simulink model "KillerWhaleModel"  (R2020b)
settings: Solver=ode15s  StartTime=0.0  StopTime=10.0  MaxStep=0.01  RelTol=1e-3
model workspace: external: MATLAB File KillerWhaleParams.m (data not in the file)
undefined symbols (not defined in the file or in its folder): frontParams, rearParams, standParams, X, Y, Z
libraries: sm_lib x4076, nesl_utility x6
(part 6 of 62)

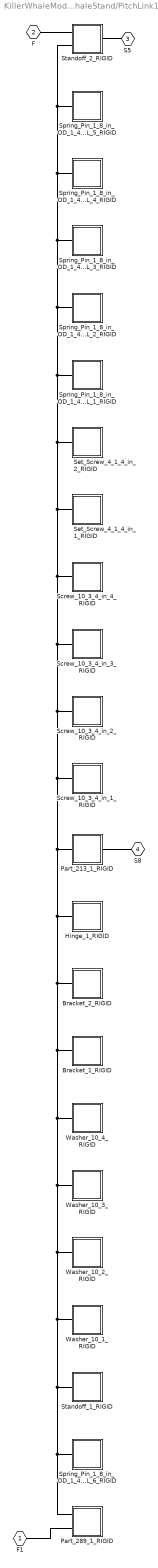
== system KillerWhaleModel/WhaleStand/PitchLink1_1 ==
  Bracket_1_RIGID : Subsystem
  Bracket_2_RIGID : Subsystem
  Hinge_1_RIGID : Subsystem
  Part_213_1_RIGID : Subsystem
  Part_289_1_RIGID : Subsystem
  Screw_10_3_4_in_1_RIGID : Subsystem
  Screw_10_3_4_in_2_RIGID : Subsystem
  Screw_10_3_4_in_3_RIGID : Subsystem
  Screw_10_3_4_in_4_RIGID : Subsystem
  Set_Screw_4_1_4_in_1_RIGID : Subsystem
  Set_Screw_4_1_4_in_2_RIGID : Subsystem
  Spring_Pin_1_8_in_OD_1_4_in_L_1_RIGID : Subsystem
  Spring_Pin_1_8_in_OD_1_4_in_L_2_RIGID : Subsystem
  Spring_Pin_1_8_in_OD_1_4_in_L_3_RIGID : Subsystem
  Spring_Pin_1_8_in_OD_1_4_in_L_4_RIGID : Subsystem
  Spring_Pin_1_8_in_OD_1_4_in_L_5_RIGID : Subsystem
  Spring_Pin_1_8_in_OD_1_4_in_L_6_RIGID : Subsystem
  Standoff_1_RIGID : Subsystem
  Standoff_2_RIGID : Subsystem
  Washer_10_1_RIGID : Subsystem
  Washer_10_2_RIGID : Subsystem
  Washer_10_3_RIGID : Subsystem
  Washer_10_4_RIGID : Subsystem
  F1 : PMIOPort  Side=Left
  F : PMIOPort  Port=2  Side=Right
  S5 : PMIOPort  Port=3  Side=Right
  S8 : PMIOPort  Port=4  Side=Right
  connections:
  Bracket_1_RIGID/LConn1 -- Part_289_1_RIGID/LConn1 -- Spring_Pin_1_8_in_OD_1_4_in_L_6_RIGID/LConn1 -- Standoff_1_RIGID/LConn1 -- Washer_10_1_RIGID/LConn1 -- Washer_10_2_RIGID/LConn1 -- Washer_10_3_RIGID/LConn1 -- Washer_10_4_RIGID/LConn1 -- Spring_Pin_1_8_in_OD_1_4_in_L_5_RIGID/LConn1 -- Standoff_2_RIGID/LConn2 -- Spring_Pin_1_8_in_OD_1_4_in_L_4_RIGID/LConn1 -- Spring_Pin_1_8_in_OD_1_4_in_L_3_RIGID/LConn1 -- Spring_Pin_1_8_in_OD_1_4_in_L_2_RIGID/LConn1 -- Spring_Pin_1_8_in_OD_1_4_in_L_1_RIGID/LConn1 -- Set_Screw_4_1_4_in_2_RIGID/LConn1 -- Set_Screw_4_1_4_in_1_RIGID/LConn1 -- Screw_10_3_4_in_4_RIGID/LConn1 -- Screw_10_3_4_in_3_RIGID/LConn1 -- Screw_10_3_4_in_2_RIGID/LConn1 -- Screw_10_3_4_in_1_RIGID/LConn1 -- Part_213_1_RIGID/LConn1 -- Hinge_1_RIGID/LConn1 -- Bracket_2_RIGID/LConn1
  Standoff_2_RIGID/LConn1 -- F/RConn1
  Part_289_1_RIGID/LConn2 -- F1/RConn1
  S5/RConn1 -- Standoff_2_RIGID/RConn1
  S8/RConn1 -- Part_213_1_RIGID/RConn1

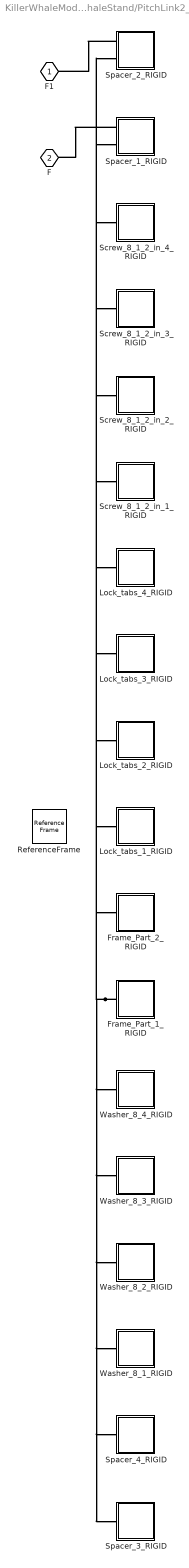
== system KillerWhaleModel/WhaleStand/PitchLink2_1 ==
  Frame_Part_1_RIGID : Subsystem
  Frame_Part_2_RIGID : Subsystem
  Lock_tabs_1_RIGID : Subsystem
  Lock_tabs_2_RIGID : Subsystem
  Lock_tabs_3_RIGID : Subsystem
  Lock_tabs_4_RIGID : Subsystem
  ReferenceFrame : sm_lib/Frames and Transforms/Reference Frame
  Screw_8_1_2_in_1_RIGID : Subsystem
  Screw_8_1_2_in_2_RIGID : Subsystem
  Screw_8_1_2_in_3_RIGID : Subsystem
  Screw_8_1_2_in_4_RIGID : Subsystem
  Spacer_1_RIGID : Subsystem
  Spacer_2_RIGID : Subsystem
  Spacer_3_RIGID : Subsystem
  Spacer_4_RIGID : Subsystem
  Washer_8_1_RIGID : Subsystem
  Washer_8_2_RIGID : Subsystem
  Washer_8_3_RIGID : Subsystem
  Washer_8_4_RIGID : Subsystem
  F1 : PMIOPort  Side=Right
  F : PMIOPort  Port=2  Side=Right
  connections:
  Frame_Part_1_RIGID/LConn1 -- Frame_Part_2_RIGID/LConn1 -- Lock_tabs_1_RIGID/LConn1 -- Lock_tabs_2_RIGID/LConn1 -- Lock_tabs_3_RIGID/LConn1 -- Lock_tabs_4_RIGID/LConn1 -- Screw_8_1_2_in_1_RIGID/LConn1 -- Screw_8_1_2_in_2_RIGID/LConn1 -- Screw_8_1_2_in_3_RIGID/LConn1 -- Screw_8_1_2_in_4_RIGID/LConn1 -- Spacer_1_RIGID/LConn2 -- Spacer_2_RIGID/LConn2 -- Spacer_3_RIGID/LConn1 -- Spacer_4_RIGID/LConn1 -- Washer_8_1_RIGID/LConn1 -- Washer_8_2_RIGID/LConn1 -- Washer_8_3_RIGID/LConn1 -- Washer_8_4_RIGID/LConn1
  Spacer_1_RIGID/LConn1 -- F/RConn1
  Spacer_2_RIGID/LConn1 -- F1/RConn1

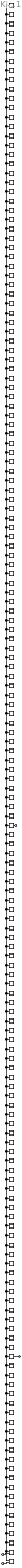
== system KillerWhaleModel/WhaleStand/PitchLink3_1 ==
  Bracket_1_RIGID : Subsystem
  Bracket_2_RIGID : Subsystem
  Bracket_3_RIGID : Subsystem
  Bracket_4_RIGID : Subsystem
  Hinge_1_RIGID : Subsystem
  Part_144_1_RIGID : Subsystem
  Part_145_1_RIGID : Subsystem
  Part_146_1_RIGID : Subsystem
  Part_147_1_RIGID : Subsystem
  Part_148_1_RIGID : Subsystem
  Part_149_1_RIGID : Subsystem
  Part_150_1_RIGID : Subsystem
  Part_151_1_RIGID : Subsystem
  Part_152_1_RIGID : Subsystem
  Part_153_1_RIGID : Subsystem
  Part_154_1_RIGID : Subsystem
  Part_155_1_RIGID : Subsystem
  Part_168_1_RIGID : Subsystem
  Part_169_1_RIGID : Subsystem
  Part_170_1_RIGID : Subsystem
  Part_171_1_RIGID : Subsystem
  Part_172_1_RIGID : Subsystem
  Part_173_1_RIGID : Subsystem
  Part_174_1_RIGID : Subsystem
  Part_175_1_RIGID : Subsystem
  Part_176_1_RIGID : Subsystem
  Part_177_1_RIGID : Subsystem
  Part_178_1_RIGID : Subsystem
  Part_179_1_RIGID : Subsystem
  Part_186_1_RIGID : Subsystem
  Part_187_1_RIGID : Subsystem
  Part_188_1_RIGID : Subsystem
  Part_190_1_RIGID : Subsystem
  Part_191_1_RIGID : Subsystem
  Part_192_1_RIGID : Subsystem
  Part_193_1_RIGID : Subsystem
  Part_194_1_RIGID : Subsystem
  Part_195_1_RIGID : Subsystem
  Part_196_1_RIGID : Subsystem
  Part_197_1_RIGID : Subsystem
  Part_318_1_RIGID : Subsystem
  Part_319_1_RIGID : Subsystem
  Part_322_1_RIGID : Subsystem
  Part_325_1_RIGID : Subsystem
  Part_328_1_RIGID : Subsystem
  Part_331_1_RIGID : Subsystem
  Part_334_1_RIGID : Subsystem
  Part_337_1_RIGID : Subsystem
  Part_340_1_RIGID : Subsystem
  Part_343_1_RIGID : Subsystem
  Part_346_1_RIGID : Subsystem
  Part_349_1_RIGID : Subsystem
  Part_360_1_RIGID : Subsystem
  Part_361_1_RIGID : Subsystem
  Part_362_1_RIGID : Subsystem
  Part_363_1_RIGID : Subsystem
  Part_364_1_RIGID : Subsystem
  Part_365_1_RIGID : Subsystem
  Part_366_1_RIGID : Subsystem
  Part_367_1_RIGID : Subsystem
  Part_368_1_RIGID : Subsystem
  Part_369_1_RIGID : Subsystem
  Part_370_1_RIGID : Subsystem
  Part_371_1_RIGID : Subsystem
  Part_372_1_RIGID : Subsystem
  Part_373_1_RIGID : Subsystem
  Part_374_1_RIGID : Subsystem
  Part_375_1_RIGID : Subsystem
  Part_380_1_RIGID : Subsystem
  Part_386_1_RIGID : Subsystem
  Part_387_1_RIGID : Subsystem
  Part_393_1_RIGID : Subsystem
  Part_399_1_RIGID : Subsystem
  Part_400_1_RIGID : Subsystem
  Part_406_1_RIGID : Subsystem
  Part_412_1_RIGID : Subsystem
  Part_413_1_RIGID : Subsystem
  Screw_10_3_4_in_10_RIGID : Subsystem
  Screw_10_3_4_in_11_RIGID : Subsystem
  Screw_10_3_4_in_12_RIGID : Subsystem
  Screw_10_3_4_in_13_RIGID : Subsystem
  Screw_10_3_4_in_14_RIGID : Subsystem
  Screw_10_3_4_in_15_RIGID : Subsystem
  Screw_10_3_4_in_16_RIGID : Subsystem
  Screw_10_3_4_in_17_RIGID : Subsystem
  Screw_10_3_4_in_18_RIGID : Subsystem
  Screw_10_3_4_in_19_RIGID : Subsystem
  Screw_10_3_4_in_1_RIGID : Subsystem
  Screw_10_3_4_in_20_RIGID : Subsystem
  Screw_10_3_4_in_2_RIGID : Subsystem
  Screw_10_3_4_in_3_RIGID : Subsystem
  Screw_10_3_4_in_4_RIGID : Subsystem
  Screw_10_3_4_in_5_RIGID : Subsystem
  Screw_10_3_4_in_6_RIGID : Subsystem
  Screw_10_3_4_in_7_RIGID : Subsystem
  Screw_10_3_4_in_8_RIGID : Subsystem
  Screw_10_3_4_in_9_RIGID : Subsystem
  Set_Screw_4_1_4_in_1_RIGID : Subsystem
  Set_Screw_4_1_4_in_2_RIGID : Subsystem
  Set_Screw_4_1_4_in_3_RIGID : Subsystem
  Set_Screw_4_1_4_in_4_RIGID : Subsystem
  Spring_Pin_1_8_in_OD_1_4_in_L_10_RIGID : Subsystem
  Spring_Pin_1_8_in_OD_1_4_in_L_11_RIGID : Subsystem
  Spring_Pin_1_8_in_OD_1_4_in_L_12_RIGID : Subsystem
  Spring_Pin_1_8_in_OD_1_4_in_L_13_RIGID : Subsystem
  Spring_Pin_1_8_in_OD_1_4_in_L_14_RIGID : Subsystem
  Spring_Pin_1_8_in_OD_1_4_in_L_15_RIGID : Subsystem
  Spring_Pin_1_8_in_OD_1_4_in_L_16_RIGID : Subsystem
  Spring_Pin_1_8_in_OD_1_4_in_L_17_RIGID : Subsystem
  Spring_Pin_1_8_in_OD_1_4_in_L_18_RIGID : Subsystem
  Spring_Pin_1_8_in_OD_1_4_in_L_19_RIGID : Subsystem
  Spring_Pin_1_8_in_OD_1_4_in_L_1_RIGID : Subsystem
  Spring_Pin_1_8_in_OD_1_4_in_L_20_RIGID : Subsystem
  Spring_Pin_1_8_in_OD_1_4_in_L_21_RIGID : Subsystem
  Spring_Pin_1_8_in_OD_1_4_in_L_22_RIGID : Subsystem
  Spring_Pin_1_8_in_OD_1_4_in_L_23_RIGID : Subsystem
  Spring_Pin_1_8_in_OD_1_4_in_L_24_RIGID : Subsystem
  Spring_Pin_1_8_in_OD_1_4_in_L_25_RIGID : Subsystem
  Spring_Pin_1_8_in_OD_1_4_in_L_26_RIGID : Subsystem
  Spring_Pin_1_8_in_OD_1_4_in_L_27_RIGID : Subsystem
  Spring_Pin_1_8_in_OD_1_4_in_L_28_RIGID : Subsystem
  Spring_Pin_1_8_in_OD_1_4_in_L_29_RIGID : Subsystem
  Spring_Pin_1_8_in_OD_1_4_in_L_2_RIGID : Subsystem
  Spring_Pin_1_8_in_OD_1_4_in_L_30_RIGID : Subsystem
  Spring_Pin_1_8_in_OD_1_4_in_L_31_RIGID : Subsystem
  Spring_Pin_1_8_in_OD_1_4_in_L_32_RIGID : Subsystem
  Spring_Pin_1_8_in_OD_1_4_in_L_33_RIGID : Subsystem
  Spring_Pin_1_8_in_OD_1_4_in_L_34_RIGID : Subsystem
  Spring_Pin_1_8_in_OD_1_4_in_L_35_RIGID : Subsystem
  Spring_Pin_1_8_in_OD_1_4_in_L_36_RIGID : Subsystem
  Spring_Pin_1_8_in_OD_1_4_in_L_37_RIGID : Subsystem
  Spring_Pin_1_8_in_OD_1_4_in_L_38_RIGID : Subsystem
  Spring_Pin_1_8_in_OD_1_4_in_L_39_RIGID : Subsystem
  Spring_Pin_1_8_in_OD_1_4_in_L_3_RIGID : Subsystem
  Spring_Pin_1_8_in_OD_1_4_in_L_40_RIGID : Subsystem
  Spring_Pin_1_8_in_OD_1_4_in_L_41_RIGID : Subsystem
  Spring_Pin_1_8_in_OD_1_4_in_L_4_RIGID : Subsystem
  Spring_Pin_1_8_in_OD_1_4_in_L_5_RIGID : Subsystem
  Spring_Pin_1_8_in_OD_1_4_in_L_6_RIGID : Subsystem
  Spring_Pin_1_8_in_OD_1_4_in_L_7_RIGID : Subsystem
  Spring_Pin_1_8_in_OD_1_4_in_L_8_RIGID : Subsystem
  Spring_Pin_1_8_in_OD_1_4_in_L_9_RIGID : Subsystem
  Washer_10_10_RIGID : Subsystem
  Washer_10_11_RIGID : Subsystem
  Washer_10_12_RIGID : Subsystem
  Washer_10_13_RIGID : Subsystem
  Washer_10_14_RIGID : Subsystem
  Washer_10_15_RIGID : Subsystem
  Washer_10_16_RIGID : Subsystem
  Washer_10_17_RIGID : Subsystem
  Washer_10_18_RIGID : Subsystem
  Washer_10_19_RIGID : Subsystem
  Washer_10_1_RIGID : Subsystem
  Washer_10_20_RIGID : Subsystem
  Washer_10_2_RIGID : Subsystem
  Washer_10_3_RIGID : Subsystem
  Washer_10_4_RIGID : Subsystem
  Washer_10_5_RIGID : Subsystem
  Washer_10_6_RIGID : Subsystem
  Washer_10_7_RIGID : Subsystem
  Washer_10_8_RIGID : Subsystem
  Washer_10_9_RIGID : Subsystem
  forward_torso_l_1_RIGID : Subsystem
  forward_torso_l_2_RIGID : Subsystem
  forward_torso_l_3_RIGID : Subsystem
  forward_torso_l_4_RIGID : Subsystem
  forward_torso_l_5_RIGID : Subsystem
  nut_1_RIGID : Subsystem
  F1 : PMIOPort  Side=Left
  S6 : PMIOPort  Port=2  Side=Left
  F : PMIOPort  Port=3  Side=Right
  S1 : PMIOPort  Port=4  Side=Right
  connections:
  Bracket_1_RIGID/LConn1 -- Part_150_1_RIGID/LConn1 -- Part_318_1_RIGID/LConn1 -- Part_346_1_RIGID/LConn1 -- Washer_10_7_RIGID/LConn1 -- Washer_10_8_RIGID/LConn1 -- Washer_10_9_RIGID/LConn1 -- forward_torso_l_1_RIGID/LConn1 -- forward_torso_l_2_RIGID/LConn1 -- forward_torso_l_3_RIGID/LConn1 -- forward_torso_l_4_RIGID/LConn1 -- forward_torso_l_5_RIGID/LConn1 -- nut_1_RIGID/LConn1 -- Washer_10_5_RIGID/LConn1 -- Washer_10_6_RIGID/LConn1 -- Washer_10_4_RIGID/LConn1 -- Washer_10_3_RIGID/LConn1 -- Washer_10_2_RIGID/LConn1 -- Washer_10_20_RIGID/LConn1 -- Washer_10_1_RIGID/LConn1 -- Washer_10_19_RIGID/LConn1 -- Washer_10_18_RIGID/LConn1 -- Washer_10_17_RIGID/LConn1 -- Washer_10_16_RIGID/LConn1 -- Washer_10_15_RIGID/LConn1 -- Washer_10_14_RIGID/LConn1 -- Washer_10_13_RIGID/LConn1 -- Washer_10_12_RIGID/LConn1 -- Washer_10_11_RIGID/LConn1 -- Washer_10_10_RIGID/LConn1 -- Spring_Pin_1_8_in_OD_1_4_in_L_9_RIGID/LConn1 -- Spring_Pin_1_8_in_OD_1_4_in_L_8_RIGID/LConn1 -- Spring_Pin_1_8_in_OD_1_4_in_L_7_RIGID/LConn1 -- Spring_Pin_1_8_in_OD_1_4_in_L_6_RIGID/LConn1 -- Spring_Pin_1_8_in_OD_1_4_in_L_5_RIGID/LConn1 -- Spring_Pin_1_8_in_OD_1_4_in_L_4_RIGID/LConn1 -- Spring_Pin_1_8_in_OD_1_4_in_L_41_RIGID/LConn1 -- Spring_Pin_1_8_in_OD_1_4_in_L_40_RIGID/LConn1 -- Spring_Pin_1_8_in_OD_1_4_in_L_3_RIGID/LConn1 -- Spring_Pin_1_8_in_OD_1_4_in_L_39_RIGID/LConn1 -- Spring_Pin_1_8_in_OD_1_4_in_L_38_RIGID/LConn1 -- Spring_Pin_1_8_in_OD_1_4_in_L_37_RIGID/LConn1 -- Spring_Pin_1_8_in_OD_1_4_in_L_36_RIGID/LConn1 -- Spring_Pin_1_8_in_OD_1_4_in_L_35_RIGID/LConn1 -- Spring_Pin_1_8_in_OD_1_4_in_L_34_RIGID/LConn1 -- Spring_Pin_1_8_in_OD_1_4_in_L_33_RIGID/LConn1 -- Spring_Pin_1_8_in_OD_1_4_in_L_32_RIGID/LConn1 -- Spring_Pin_1_8_in_OD_1_4_in_L_31_RIGID/LConn1 -- Spring_Pin_1_8_in_OD_1_4_in_L_30_RIGID/LConn1 -- Spring_Pin_1_8_in_OD_1_4_in_L_2_RIGID/LConn1 -- Spring_Pin_1_8_in_OD_1_4_in_L_29_RIGID/LConn1 -- Spring_Pin_1_8_in_OD_1_4_in_L_28_RIGID/LConn1 -- Spring_Pin_1_8_in_OD_1_4_in_L_27_RIGID/LConn1 -- Spring_Pin_1_8_in_OD_1_4_in_L_26_RIGID/LConn1 -- Spring_Pin_1_8_in_OD_1_4_in_L_25_RIGID/LConn1 -- Spring_Pin_1_8_in_OD_1_4_in_L_24_RIGID/LConn1 -- Spring_Pin_1_8_in_OD_1_4_in_L_23_RIGID/LConn1 -- Spring_Pin_1_8_in_OD_1_4_in_L_22_RIGID/LConn1 -- Spring_Pin_1_8_in_OD_1_4_in_L_21_RIGID/LConn1 -- Spring_Pin_1_8_in_OD_1_4_in_L_20_RIGID/LConn1 -- Spring_Pin_1_8_in_OD_1_4_in_L_1_RIGID/LConn1 -- Spring_Pin_1_8_in_OD_1_4_in_L_19_RIGID/LConn1 -- Spring_Pin_1_8_in_OD_1_4_in_L_18_RIGID/LConn1 -- Spring_Pin_1_8_in_OD_1_4_in_L_17_RIGID/LConn1 -- Spring_Pin_1_8_in_OD_1_4_in_L_16_RIGID/LConn1 -- Spring_Pin_1_8_in_OD_1_4_in_L_15_RIGID/LConn1 -- Spring_Pin_1_8_in_OD_1_4_in_L_14_RIGID/LConn1 -- Spring_Pin_1_8_in_OD_1_4_in_L_13_RIGID/LConn1 -- Spring_Pin_1_8_in_OD_1_4_in_L_12_RIGID/LConn1 -- Spring_Pin_1_8_in_OD_1_4_in_L_11_RIGID/LConn1 -- Spring_Pin_1_8_in_OD_1_4_in_L_10_RIGID/LConn1 -- Set_Screw_4_1_4_in_4_RIGID/LConn1 -- Set_Screw_4_1_4_in_3_RIGID/LConn1 -- Set_Screw_4_1_4_in_2_RIGID/LConn1 -- Set_Screw_4_1_4_in_1_RIGID/LConn1 -- Screw_10_3_4_in_9_RIGID/LConn1 -- Screw_10_3_4_in_8_RIGID/LConn1 -- Screw_10_3_4_in_7_RIGID/LConn1 -- Screw_10_3_4_in_6_RIGID/LConn1 -- Screw_10_3_4_in_5_RIGID/LConn1 -- Screw_10_3_4_in_4_RIGID/LConn1 -- Screw_10_3_4_in_3_RIGID/LConn1 -- Screw_10_3_4_in_2_RIGID/LConn1 -- Screw_10_3_4_in_20_RIGID/LConn1 -- Screw_10_3_4_in_1_RIGID/LConn1 -- Screw_10_3_4_in_19_RIGID/LConn1 -- Screw_10_3_4_in_18_RIGID/LConn1 -- Screw_10_3_4_in_17_RIGID/LConn1 -- Screw_10_3_4_in_16_RIGID/LConn1 -- Screw_10_3_4_in_15_RIGID/LConn1 -- Screw_10_3_4_in_14_RIGID/LConn1 -- Screw_10_3_4_in_13_RIGID/LConn1 -- Screw_10_3_4_in_12_RIGID/LConn1 -- Screw_10_3_4_in_11_RIGID/LConn1 -- Screw_10_3_4_in_10_RIGID/LConn1 -- Part_413_1_RIGID/LConn1 -- Part_412_1_RIGID/LConn1 -- Part_406_1_RIGID/LConn1 -- Part_400_1_RIGID/LConn1 -- Part_399_1_RIGID/LConn1 -- Part_393_1_RIGID/LConn1 -- Part_387_1_RIGID/LConn1 -- Part_386_1_RIGID/LConn1 -- Part_380_1_RIGID/LConn1 -- Part_375_1_RIGID/LConn1 -- Part_374_1_RIGID/LConn1 -- Part_373_1_RIGID/LConn1 -- Part_372_1_RIGID/LConn1 -- Part_371_1_RIGID/LConn1 -- Part_370_1_RIGID/LConn1 -- Part_369_1_RIGID/LConn1 -- Part_368_1_RIGID/LConn1 -- Part_367_1_RIGID/LConn1 -- Part_366_1_RIGID/LConn1 -- Part_365_1_RIGID/LConn1 -- Part_364_1_RIGID/LConn1 -- Part_363_1_RIGID/LConn1 -- Part_362_1_RIGID/LConn1 -- Part_361_1_RIGID/LConn1 -- Part_360_1_RIGID/LConn1 -- Part_349_1_RIGID/LConn1 -- Part_343_1_RIGID/LConn1 -- Part_340_1_RIGID/LConn1 -- Part_337_1_RIGID/LConn1 -- Part_334_1_RIGID/LConn1 -- Part_331_1_RIGID/LConn1 -- Part_328_1_RIGID/LConn1 -- Part_325_1_RIGID/LConn1 -- Part_322_1_RIGID/LConn1 -- Part_319_1_RIGID/LConn1 -- Part_197_1_RIGID/LConn1 -- Part_196_1_RIGID/LConn1 -- Part_195_1_RIGID/LConn1 -- Part_194_1_RIGID/LConn1 -- Part_193_1_RIGID/LConn1 -- Part_192_1_RIGID/LConn1 -- Part_191_1_RIGID/LConn1 -- Part_190_1_RIGID/LConn1 -- Part_188_1_RIGID/LConn1 -- Part_187_1_RIGID/LConn1 -- Part_186_1_RIGID/LConn1 -- Part_179_1_RIGID/LConn1 -- Part_178_1_RIGID/LConn1 -- Part_177_1_RIGID/LConn1 -- Part_176_1_RIGID/LConn1 -- Part_175_1_RIGID/LConn1 -- Part_174_1_RIGID/LConn1 -- Part_173_1_RIGID/LConn1 -- Part_172_1_RIGID/LConn1 -- Part_171_1_RIGID/LConn1 -- Part_170_1_RIGID/LConn1 -- Part_169_1_RIGID/LConn1 -- Part_168_1_RIGID/LConn1 -- Part_155_1_RIGID/LConn1 -- Part_154_1_RIGID/LConn1 -- Part_153_1_RIGID/LConn1 -- Part_152_1_RIGID/LConn1 -- Part_151_1_RIGID/LConn1 -- Part_149_1_RIGID/LConn1 -- Part_148_1_RIGID/LConn1 -- Part_147_1_RIGID/LConn1 -- Part_146_1_RIGID/LConn1 -- Part_145_1_RIGID/LConn1 -- Part_144_1_RIGID/LConn1 -- Hinge_1_RIGID/LConn1 -- Bracket_4_RIGID/LConn1 -- Bracket_3_RIGID/LConn1 -- Bracket_2_RIGID/LConn1
  Part_150_1_RIGID/LConn2 -- F/RConn1
  Part_318_1_RIGID/LConn2 -- F1/RConn1
  S1/RConn1 -- Part_149_1_RIGID/RConn1
  S6/RConn1 -- Part_387_1_RIGID/RConn1

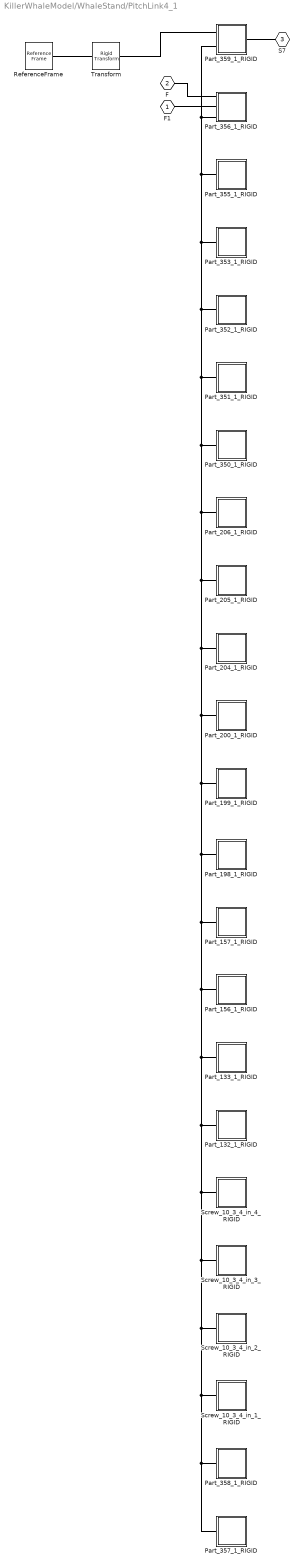
== system KillerWhaleModel/WhaleStand/PitchLink4_1 ==
  Part_132_1_RIGID : Subsystem
  Part_133_1_RIGID : Subsystem
  Part_156_1_RIGID : Subsystem
  Part_157_1_RIGID : Subsystem
  Part_198_1_RIGID : Subsystem
  Part_199_1_RIGID : Subsystem
  Part_200_1_RIGID : Subsystem
  Part_204_1_RIGID : Subsystem
  Part_205_1_RIGID : Subsystem
  Part_206_1_RIGID : Subsystem
  Part_350_1_RIGID : Subsystem
  Part_351_1_RIGID : Subsystem
  Part_352_1_RIGID : Subsystem
  Part_353_1_RIGID : Subsystem
  Part_355_1_RIGID : Subsystem
  Part_356_1_RIGID : Subsystem
  Part_357_1_RIGID : Subsystem
  Part_358_1_RIGID : Subsystem
  Part_359_1_RIGID : Subsystem
  ReferenceFrame : sm_lib/Frames and Transforms/Reference Frame
  Screw_10_3_4_in_1_RIGID : Subsystem
  Screw_10_3_4_in_2_RIGID : Subsystem
  Screw_10_3_4_in_3_RIGID : Subsystem
  Screw_10_3_4_in_4_RIGID : Subsystem
  Transform : sm_lib/Frames and Transforms/Rigid Transform  TranslationMethod=Cartesian  TranslationStandardOffset=0  TranslationLengthUnit=in  TranslationStandardAxis=+Z  TranslationCartesianOffset=standParams.RigidTransform(241).translation  TranslationROffset=0  TranslationROffsetUnits=m  TranslationZOffset=0  TranslationZOffsetUnits=m  TranslationThetaOffset=0  TranslationThetaOffsetUnits=deg  RotationMethod=ArbitraryAxis  RotationAngleUnits=rad  RotationStandardAxis=+Z  RotationAngle=standParams.RigidTransform(241).angle  RotationArbitraryAxis=standParams.RigidTransform(241).axis  FollAlignAxisA=+X  BaseAlignAxisA=+Y  FollAlignAxisB=+Y  BaseAlignAxisB=+Z  RotationSequenceAxes=FollowerAxes  RotationSequence=XYX  RotationSequenceAngles=[0 0 0]  RotationSequenceAnglesUnits=deg  RotationMatrix=[1 0 0; 0 1 0; 0 0 1]
  F1 : PMIOPort  Side=Left
  F : PMIOPort  Port=2  Side=Left
  S7 : PMIOPort  Port=3  Side=Right
  connections:
  Part_132_1_RIGID/LConn1 -- Part_357_1_RIGID/LConn1 -- Part_358_1_RIGID/LConn1 -- Screw_10_3_4_in_1_RIGID/LConn1 -- Screw_10_3_4_in_2_RIGID/LConn1 -- Screw_10_3_4_in_3_RIGID/LConn1 -- Screw_10_3_4_in_4_RIGID/LConn1 -- Part_356_1_RIGID/LConn3 -- Part_359_1_RIGID/LConn2 -- Part_355_1_RIGID/LConn1 -- Part_353_1_RIGID/LConn1 -- Part_352_1_RIGID/LConn1 -- Part_351_1_RIGID/LConn1 -- Part_350_1_RIGID/LConn1 -- Part_206_1_RIGID/LConn1 -- Part_205_1_RIGID/LConn1 -- Part_204_1_RIGID/LConn1 -- Part_200_1_RIGID/LConn1 -- Part_199_1_RIGID/LConn1 -- Part_198_1_RIGID/LConn1 -- Part_157_1_RIGID/LConn1 -- Part_156_1_RIGID/LConn1 -- Part_133_1_RIGID/LConn1
  Part_356_1_RIGID/LConn1 -- F/RConn1
  Part_356_1_RIGID/LConn2 -- F1/RConn1
  Part_359_1_RIGID/LConn1 -- Transform/RConn1
  ReferenceFrame/RConn1 -- Transform/LConn1
  S7/RConn1 -- Part_359_1_RIGID/RConn1

== system KillerWhaleModel/HeadLinkage/HeadLink1_1/Bracket_1_RIGID ==
  ReferenceFrame : sm_lib/Frames and Transforms/Reference Frame
  Solid : sm_lib/Body Elements/File Solid  ExtGeomFileName=Bracket13.step  UnitType=FromFile  ExtGeomFileUnits=m  StepReaderType=HEX  ExportConvexHullGeometry=off  InertiaType=Custom  Mass=frontParams.Solid(20).mass  MassUnits=lbm  CenterOfMass=frontParams.Solid(20).CoM  CenterOfMassUnits=in  MomentsOfInertia=frontParams.Solid(20).MoI  MomentsOfInertiaUnits=lbm*in^2  ProductsOfInertia=frontParams.Solid(20).PoI  ProductsOfInertiaUnits=lbm*in^2  BasedOnType=DensityFromFile  Density=1000  DensityUnits=kg/m^3  DoExposeReferenceFrame=on  SerializedFrames=<Frames/>  GraphicType=FromGeometry  MarkerShape=Sphere  MarkerSize=10  GraphicVisPropType=SimpleVisualProperties  GraphicDiffuseColor=frontParams.Solid(20).color  GraphicSpecularColor=[0.5 0.5 0.5 1.0]  GraphicAmbientColor=[0.15 0.15 0.15 1.0]  GraphicEmissiveColor=[0.0 0.0 0.0 1.0]  GraphicShininess=75  GraphicOpacity=frontParams.Solid(20).opacity
  Transform : sm_lib/Frames and Transforms/Rigid Transform  TranslationMethod=Cartesian  TranslationStandardOffset=0  TranslationLengthUnit=in  TranslationStandardAxis=+Z  TranslationCartesianOffset=frontParams.RigidTransform(33).translation  TranslationROffset=0  TranslationROffsetUnits=m  TranslationZOffset=0  TranslationZOffsetUnits=m  TranslationThetaOffset=0  TranslationThetaOffsetUnits=deg  RotationMethod=ArbitraryAxis  RotationAngleUnits=rad  RotationStandardAxis=+Z  RotationAngle=frontParams.RigidTransform(33).angle  RotationArbitraryAxis=frontParams.RigidTransform(33).axis  FollAlignAxisA=+X  BaseAlignAxisA=+Y  FollAlignAxisB=+Y  BaseAlignAxisB=+Z  RotationSequenceAxes=FollowerAxes  RotationSequence=XYX  RotationSequenceAngles=[0 0 0]  RotationSequenceAnglesUnits=deg  RotationMatrix=[1 0 0; 0 1 0; 0 0 1]
  G : PMIOPort  Side=Left
  connections:
  ReferenceFrame/RConn1 -- Solid/RConn1 -- Transform/RConn1
  Transform/LConn1 -- G/RConn1

== system KillerWhaleModel/HeadLinkage/HeadLink1_1/Bracket_2_RIGID ==
  ReferenceFrame : sm_lib/Frames and Transforms/Reference Frame
  Solid : sm_lib/Body Elements/File Solid  ExtGeomFileName=Bracket14.step  UnitType=FromFile  ExtGeomFileUnits=m  StepReaderType=HEX  ExportConvexHullGeometry=off  InertiaType=Custom  Mass=frontParams.Solid(52).mass  MassUnits=lbm  CenterOfMass=frontParams.Solid(52).CoM  CenterOfMassUnits=in  MomentsOfInertia=frontParams.Solid(52).MoI  MomentsOfInertiaUnits=lbm*in^2  ProductsOfInertia=frontParams.Solid(52).PoI  ProductsOfInertiaUnits=lbm*in^2  BasedOnType=DensityFromFile  Density=1000  DensityUnits=kg/m^3  DoExposeReferenceFrame=on  SerializedFrames=<Frames/>  GraphicType=FromGeometry  MarkerShape=Sphere  MarkerSize=10  GraphicVisPropType=SimpleVisualProperties  GraphicDiffuseColor=frontParams.Solid(52).color  GraphicSpecularColor=[0.5 0.5 0.5 1.0]  GraphicAmbientColor=[0.15 0.15 0.15 1.0]  GraphicEmissiveColor=[0.0 0.0 0.0 1.0]  GraphicShininess=75  GraphicOpacity=frontParams.Solid(52).opacity
  Transform : sm_lib/Frames and Transforms/Rigid Transform  TranslationMethod=Cartesian  TranslationStandardOffset=0  TranslationLengthUnit=in  TranslationStandardAxis=+Z  TranslationCartesianOffset=frontParams.RigidTransform(65).translation  TranslationROffset=0  TranslationROffsetUnits=m  TranslationZOffset=0  TranslationZOffsetUnits=m  TranslationThetaOffset=0  TranslationThetaOffsetUnits=deg  RotationMethod=ArbitraryAxis  RotationAngleUnits=rad  RotationStandardAxis=+Z  RotationAngle=frontParams.RigidTransform(65).angle  RotationArbitraryAxis=frontParams.RigidTransform(65).axis  FollAlignAxisA=+X  BaseAlignAxisA=+Y  FollAlignAxisB=+Y  BaseAlignAxisB=+Z  RotationSequenceAxes=FollowerAxes  RotationSequence=XYX  RotationSequenceAngles=[0 0 0]  RotationSequenceAnglesUnits=deg  RotationMatrix=[1 0 0; 0 1 0; 0 0 1]
  G : PMIOPort  Side=Left
  connections:
  ReferenceFrame/RConn1 -- Solid/RConn1 -- Transform/RConn1
  Transform/LConn1 -- G/RConn1

== system KillerWhaleModel/HeadLinkage/HeadLink1_1/Hinge_1_RIGID ==
  ReferenceFrame : sm_lib/Frames and Transforms/Reference Frame
  Solid : sm_lib/Body Elements/File Solid  ExtGeomFileName=Hinge6.step  UnitType=FromFile  ExtGeomFileUnits=m  StepReaderType=HEX  ExportConvexHullGeometry=off  InertiaType=Custom  Mass=frontParams.Solid(3).mass  MassUnits=lbm  CenterOfMass=frontParams.Solid(3).CoM  CenterOfMassUnits=in  MomentsOfInertia=frontParams.Solid(3).MoI  MomentsOfInertiaUnits=lbm*in^2  ProductsOfInertia=frontParams.Solid(3).PoI  ProductsOfInertiaUnits=lbm*in^2  BasedOnType=DensityFromFile  Density=1000  DensityUnits=kg/m^3  DoExposeReferenceFrame=on  SerializedFrames=<Frames/>  GraphicType=FromGeometry  MarkerShape=Sphere  MarkerSize=10  GraphicVisPropType=SimpleVisualProperties  GraphicDiffuseColor=frontParams.Solid(3).color  GraphicSpecularColor=[0.5 0.5 0.5 1.0]  GraphicAmbientColor=[0.15 0.15 0.15 1.0]  GraphicEmissiveColor=[0.0 0.0 0.0 1.0]  GraphicShininess=75  GraphicOpacity=frontParams.Solid(3).opacity
  Transform : sm_lib/Frames and Transforms/Rigid Transform  TranslationMethod=Cartesian  TranslationStandardOffset=0  TranslationLengthUnit=in  TranslationStandardAxis=+Z  TranslationCartesianOffset=frontParams.RigidTransform(16).translation  TranslationROffset=0  TranslationROffsetUnits=m  TranslationZOffset=0  TranslationZOffsetUnits=m  TranslationThetaOffset=0  TranslationThetaOffsetUnits=deg  RotationMethod=ArbitraryAxis  RotationAngleUnits=rad  RotationStandardAxis=+Z  RotationAngle=frontParams.RigidTransform(16).angle  RotationArbitraryAxis=frontParams.RigidTransform(16).axis  FollAlignAxisA=+X  BaseAlignAxisA=+Y  FollAlignAxisB=+Y  BaseAlignAxisB=+Z  RotationSequenceAxes=FollowerAxes  RotationSequence=XYX  RotationSequenceAngles=[0 0 0]  RotationSequenceAnglesUnits=deg  RotationMatrix=[1 0 0; 0 1 0; 0 0 1]
  G : PMIOPort  Side=Left
  connections:
  ReferenceFrame/RConn1 -- Solid/RConn1 -- Transform/RConn1
  Transform/LConn1 -- G/RConn1

== system KillerWhaleModel/HeadLinkage/HeadLink1_1/Part_1_1_RIGID ==
  ReferenceFrame : sm_lib/Frames and Transforms/Reference Frame
  Solid : sm_lib/Body Elements/File Solid  ExtGeomFileName=Part 111.step  UnitType=FromFile  ExtGeomFileUnits=m  StepReaderType=HEX  ExportConvexHullGeometry=off  InertiaType=Custom  Mass=frontParams.Solid(50).mass  MassUnits=lbm  CenterOfMass=frontParams.Solid(50).CoM  CenterOfMassUnits=in  MomentsOfInertia=frontParams.Solid(50).MoI  MomentsOfInertiaUnits=lbm*in^2  ProductsOfInertia=frontParams.Solid(50).PoI  ProductsOfInertiaUnits=lbm*in^2  BasedOnType=DensityFromFile  Density=1000  DensityUnits=kg/m^3  DoExposeReferenceFrame=on  SerializedFrames=<Frames/>  GraphicType=FromGeometry  MarkerShape=Sphere  MarkerSize=10  GraphicVisPropType=SimpleVisualProperties  GraphicDiffuseColor=frontParams.Solid(50).color  GraphicSpecularColor=[0.5 0.5 0.5 1.0]  GraphicAmbientColor=[0.15 0.15 0.15 1.0]  GraphicEmissiveColor=[0.0 0.0 0.0 1.0]  GraphicShininess=75  GraphicOpacity=frontParams.Solid(50).opacity
  Transform : sm_lib/Frames and Transforms/Rigid Transform  TranslationMethod=Cartesian  TranslationStandardOffset=0  TranslationLengthUnit=in  TranslationStandardAxis=+Z  TranslationCartesianOffset=frontParams.RigidTransform(63).translation  TranslationROffset=0  TranslationROffsetUnits=m  TranslationZOffset=0  TranslationZOffsetUnits=m  TranslationThetaOffset=0  TranslationThetaOffsetUnits=deg  RotationMethod=ArbitraryAxis  RotationAngleUnits=rad  RotationStandardAxis=+Z  RotationAngle=frontParams.RigidTransform(63).angle  RotationArbitraryAxis=frontParams.RigidTransform(63).axis  FollAlignAxisA=+X  BaseAlignAxisA=+Y  FollAlignAxisB=+Y  BaseAlignAxisB=+Z  RotationSequenceAxes=FollowerAxes  RotationSequence=XYX  RotationSequenceAngles=[0 0 0]  RotationSequenceAnglesUnits=deg  RotationMatrix=[1 0 0; 0 1 0; 0 0 1]
  G : PMIOPort  Side=Left
  connections:
  ReferenceFrame/RConn1 -- Solid/RConn1 -- Transform/RConn1
  Transform/LConn1 -- G/RConn1

== system KillerWhaleModel/HeadLinkage/HeadLink1_1/Part_1_2_RIGID ==
  ReferenceFrame : sm_lib/Frames and Transforms/Reference Frame
  Solid : sm_lib/Body Elements/File Solid  ExtGeomFileName=Part 110.step  UnitType=FromFile  ExtGeomFileUnits=m  StepReaderType=HEX  ExportConvexHullGeometry=off  InertiaType=Custom  Mass=frontParams.Solid(12).mass  MassUnits=lbm  CenterOfMass=frontParams.Solid(12).CoM  CenterOfMassUnits=in  MomentsOfInertia=frontParams.Solid(12).MoI  MomentsOfInertiaUnits=lbm*in^2  ProductsOfInertia=frontParams.Solid(12).PoI  ProductsOfInertiaUnits=lbm*in^2  BasedOnType=DensityFromFile  Density=1000  DensityUnits=kg/m^3  DoExposeReferenceFrame=on  SerializedFrames=<Frames/>  GraphicType=FromGeometry  MarkerShape=Sphere  MarkerSize=10  GraphicVisPropType=SimpleVisualProperties  GraphicDiffuseColor=frontParams.Solid(12).color  GraphicSpecularColor=[0.5 0.5 0.5 1.0]  GraphicAmbientColor=[0.15 0.15 0.15 1.0]  GraphicEmissiveColor=[0.0 0.0 0.0 1.0]  GraphicShininess=75  GraphicOpacity=frontParams.Solid(12).opacity
  Transform : sm_lib/Frames and Transforms/Rigid Transform  TranslationMethod=Cartesian  TranslationStandardOffset=0  TranslationLengthUnit=in  TranslationStandardAxis=+Z  TranslationCartesianOffset=frontParams.RigidTransform(25).translation  TranslationROffset=0  TranslationROffsetUnits=m  TranslationZOffset=0  TranslationZOffsetUnits=m  TranslationThetaOffset=0  TranslationThetaOffsetUnits=deg  RotationMethod=ArbitraryAxis  RotationAngleUnits=rad  RotationStandardAxis=+Z  RotationAngle=frontParams.RigidTransform(25).angle  RotationArbitraryAxis=frontParams.RigidTransform(25).axis  FollAlignAxisA=+X  BaseAlignAxisA=+Y  FollAlignAxisB=+Y  BaseAlignAxisB=+Z  RotationSequenceAxes=FollowerAxes  RotationSequence=XYX  RotationSequenceAngles=[0 0 0]  RotationSequenceAnglesUnits=deg  RotationMatrix=[1 0 0; 0 1 0; 0 0 1]
  G : PMIOPort  Side=Left
  connections:
  ReferenceFrame/RConn1 -- Solid/RConn1 -- Transform/RConn1
  Transform/LConn1 -- G/RConn1

== system KillerWhaleModel/HeadLinkage/HeadLink1_1/Part_2_1_RIGID ==
  ReferenceFrame : sm_lib/Frames and Transforms/Reference Frame
  Solid : sm_lib/Body Elements/File Solid  ExtGeomFileName=Part 28.step  UnitType=FromFile  ExtGeomFileUnits=m  StepReaderType=HEX  ExportConvexHullGeometry=off  InertiaType=Custom  Mass=frontParams.Solid(36).mass  MassUnits=lbm  CenterOfMass=frontParams.Solid(36).CoM  CenterOfMassUnits=in  MomentsOfInertia=frontParams.Solid(36).MoI  MomentsOfInertiaUnits=lbm*in^2  ProductsOfInertia=frontParams.Solid(36).PoI  ProductsOfInertiaUnits=lbm*in^2  BasedOnType=DensityFromFile  Density=1000  DensityUnits=kg/m^3  DoExposeReferenceFrame=on  SerializedFrames=<Frames/>  GraphicType=FromGeometry  MarkerShape=Sphere  MarkerSize=10  GraphicVisPropType=SimpleVisualProperties  GraphicDiffuseColor=frontParams.Solid(36).color  GraphicSpecularColor=[0.5 0.5 0.5 1.0]  GraphicAmbientColor=[0.15 0.15 0.15 1.0]  GraphicEmissiveColor=[0.0 0.0 0.0 1.0]  GraphicShininess=75  GraphicOpacity=frontParams.Solid(36).opacity
  Transform : sm_lib/Frames and Transforms/Rigid Transform  TranslationMethod=Cartesian  TranslationStandardOffset=0  TranslationLengthUnit=in  TranslationStandardAxis=+Z  TranslationCartesianOffset=frontParams.RigidTransform(49).translation  TranslationROffset=0  TranslationROffsetUnits=m  TranslationZOffset=0  TranslationZOffsetUnits=m  TranslationThetaOffset=0  TranslationThetaOffsetUnits=deg  RotationMethod=ArbitraryAxis  RotationAngleUnits=rad  RotationStandardAxis=+Z  RotationAngle=frontParams.RigidTransform(49).angle  RotationArbitraryAxis=frontParams.RigidTransform(49).axis  FollAlignAxisA=+X  BaseAlignAxisA=+Y  FollAlignAxisB=+Y  BaseAlignAxisB=+Z  RotationSequenceAxes=FollowerAxes  RotationSequence=XYX  RotationSequenceAngles=[0 0 0]  RotationSequenceAnglesUnits=deg  RotationMatrix=[1 0 0; 0 1 0; 0 0 1]
  G : PMIOPort  Side=Left
  connections:
  ReferenceFrame/RConn1 -- Solid/RConn1 -- Transform/RConn1
  Transform/LConn1 -- G/RConn1

== system KillerWhaleModel/HeadLinkage/HeadLink1_1/Part_2_2_RIGID ==
  ReferenceFrame : sm_lib/Frames and Transforms/Reference Frame
  Solid : sm_lib/Body Elements/File Solid  ExtGeomFileName=Part 27.step  UnitType=FromFile  ExtGeomFileUnits=m  StepReaderType=HEX  ExportConvexHullGeometry=off  InertiaType=Custom  Mass=frontParams.Solid(51).mass  MassUnits=lbm  CenterOfMass=frontParams.Solid(51).CoM  CenterOfMassUnits=in  MomentsOfInertia=frontParams.Solid(51).MoI  MomentsOfInertiaUnits=lbm*in^2  ProductsOfInertia=frontParams.Solid(51).PoI  ProductsOfInertiaUnits=lbm*in^2  BasedOnType=DensityFromFile  Density=1000  DensityUnits=kg/m^3  DoExposeReferenceFrame=on  SerializedFrames=<Frames/>  GraphicType=FromGeometry  MarkerShape=Sphere  MarkerSize=10  GraphicVisPropType=SimpleVisualProperties  GraphicDiffuseColor=frontParams.Solid(51).color  GraphicSpecularColor=[0.5 0.5 0.5 1.0]  GraphicAmbientColor=[0.15 0.15 0.15 1.0]  GraphicEmissiveColor=[0.0 0.0 0.0 1.0]  GraphicShininess=75  GraphicOpacity=frontParams.Solid(51).opacity
  Transform : sm_lib/Frames and Transforms/Rigid Transform  TranslationMethod=Cartesian  TranslationStandardOffset=0  TranslationLengthUnit=in  TranslationStandardAxis=+Z  TranslationCartesianOffset=frontParams.RigidTransform(64).translation  TranslationROffset=0  TranslationROffsetUnits=m  TranslationZOffset=0  TranslationZOffsetUnits=m  TranslationThetaOffset=0  TranslationThetaOffsetUnits=deg  RotationMethod=ArbitraryAxis  RotationAngleUnits=rad  RotationStandardAxis=+Z  RotationAngle=frontParams.RigidTransform(64).angle  RotationArbitraryAxis=frontParams.RigidTransform(64).axis  FollAlignAxisA=+X  BaseAlignAxisA=+Y  FollAlignAxisB=+Y  BaseAlignAxisB=+Z  RotationSequenceAxes=FollowerAxes  RotationSequence=XYX  RotationSequenceAngles=[0 0 0]  RotationSequenceAnglesUnits=deg  RotationMatrix=[1 0 0; 0 1 0; 0 0 1]
  G : PMIOPort  Side=Left
  connections:
  ReferenceFrame/RConn1 -- Solid/RConn1 -- Transform/RConn1
  Transform/LConn1 -- G/RConn1

== system KillerWhaleModel/HeadLinkage/HeadLink1_1/Part_3_1_RIGID ==
  ReferenceFrame : sm_lib/Frames and Transforms/Reference Frame
  Solid : sm_lib/Body Elements/File Solid  ExtGeomFileName=Part 31.step  UnitType=FromFile  ExtGeomFileUnits=m  StepReaderType=HEX  ExportConvexHullGeometry=off  InertiaType=Custom  Mass=frontParams.Solid(55).mass  MassUnits=lbm  CenterOfMass=frontParams.Solid(55).CoM  CenterOfMassUnits=in  MomentsOfInertia=frontParams.Solid(55).MoI  MomentsOfInertiaUnits=lbm*in^2  ProductsOfInertia=frontParams.Solid(55).PoI  ProductsOfInertiaUnits=lbm*in^2  BasedOnType=DensityFromFile  Density=1000  DensityUnits=kg/m^3  DoExposeReferenceFrame=on  SerializedFrames=<Frames/>  GraphicType=FromGeometry  MarkerShape=Sphere  MarkerSize=10  GraphicVisPropType=SimpleVisualProperties  GraphicDiffuseColor=frontParams.Solid(55).color  GraphicSpecularColor=[0.5 0.5 0.5 1.0]  GraphicAmbientColor=[0.15 0.15 0.15 1.0]  GraphicEmissiveColor=[0.0 0.0 0.0 1.0]  GraphicShininess=75  GraphicOpacity=frontParams.Solid(55).opacity
  Transform : sm_lib/Frames and Transforms/Rigid Transform  TranslationMethod=Cartesian  TranslationStandardOffset=0  TranslationLengthUnit=in  TranslationStandardAxis=+Z  TranslationCartesianOffset=frontParams.RigidTransform(68).translation  TranslationROffset=0  TranslationROffsetUnits=m  TranslationZOffset=0  TranslationZOffsetUnits=m  TranslationThetaOffset=0  TranslationThetaOffsetUnits=deg  RotationMethod=ArbitraryAxis  RotationAngleUnits=rad  RotationStandardAxis=+Z  RotationAngle=frontParams.RigidTransform(68).angle  RotationArbitraryAxis=frontParams.RigidTransform(68).axis  FollAlignAxisA=+X  BaseAlignAxisA=+Y  FollAlignAxisB=+Y  BaseAlignAxisB=+Z  RotationSequenceAxes=FollowerAxes  RotationSequence=XYX  RotationSequenceAngles=[0 0 0]  RotationSequenceAnglesUnits=deg  RotationMatrix=[1 0 0; 0 1 0; 0 0 1]
  G : PMIOPort  Side=Left
  connections:
  ReferenceFrame/RConn1 -- Solid/RConn1 -- Transform/RConn1
  Transform/LConn1 -- G/RConn1

== system KillerWhaleModel/HeadLinkage/HeadLink1_1/Part_3_2_RIGID ==
  ReferenceFrame : sm_lib/Frames and Transforms/Reference Frame
  Solid : sm_lib/Body Elements/File Solid  ExtGeomFileName=Part 32.step  UnitType=FromFile  ExtGeomFileUnits=m  StepReaderType=HEX  ExportConvexHullGeometry=off  InertiaType=Custom  Mass=frontParams.Solid(17).mass  MassUnits=lbm  CenterOfMass=frontParams.Solid(17).CoM  CenterOfMassUnits=in  MomentsOfInertia=frontParams.Solid(17).MoI  MomentsOfInertiaUnits=lbm*in^2  ProductsOfInertia=frontParams.Solid(17).PoI  ProductsOfInertiaUnits=lbm*in^2  BasedOnType=DensityFromFile  Density=1000  DensityUnits=kg/m^3  DoExposeReferenceFrame=on  SerializedFrames=<Frames/>  GraphicType=FromGeometry  MarkerShape=Sphere  MarkerSize=10  GraphicVisPropType=SimpleVisualProperties  GraphicDiffuseColor=frontParams.Solid(17).color  GraphicSpecularColor=[0.5 0.5 0.5 1.0]  GraphicAmbientColor=[0.15 0.15 0.15 1.0]  GraphicEmissiveColor=[0.0 0.0 0.0 1.0]  GraphicShininess=75  GraphicOpacity=frontParams.Solid(17).opacity
  Transform : sm_lib/Frames and Transforms/Rigid Transform  TranslationMethod=Cartesian  TranslationStandardOffset=0  TranslationLengthUnit=in  TranslationStandardAxis=+Z  TranslationCartesianOffset=frontParams.RigidTransform(30).translation  TranslationROffset=0  TranslationROffsetUnits=m  TranslationZOffset=0  TranslationZOffsetUnits=m  TranslationThetaOffset=0  TranslationThetaOffsetUnits=deg  RotationMethod=ArbitraryAxis  RotationAngleUnits=rad  RotationStandardAxis=+Z  RotationAngle=frontParams.RigidTransform(30).angle  RotationArbitraryAxis=frontParams.RigidTransform(30).axis  FollAlignAxisA=+X  BaseAlignAxisA=+Y  FollAlignAxisB=+Y  BaseAlignAxisB=+Z  RotationSequenceAxes=FollowerAxes  RotationSequence=XYX  RotationSequenceAngles=[0 0 0]  RotationSequenceAnglesUnits=deg  RotationMatrix=[1 0 0; 0 1 0; 0 0 1]
  G : PMIOPort  Side=Left
  connections:
  ReferenceFrame/RConn1 -- Solid/RConn1 -- Transform/RConn1
  Transform/LConn1 -- G/RConn1

== system KillerWhaleModel/HeadLinkage/HeadLink1_1/Part_40_1_RIGID ==
  ReferenceFrame : sm_lib/Frames and Transforms/Reference Frame
  Solid : sm_lib/Body Elements/File Solid  ExtGeomFileName=Part 40.step  UnitType=FromFile  ExtGeomFileUnits=m  StepReaderType=HEX  ExportConvexHullGeometry=off  InertiaType=Custom  Mass=frontParams.Solid(27).mass  MassUnits=lbm  CenterOfMass=frontParams.Solid(27).CoM  CenterOfMassUnits=in  MomentsOfInertia=frontParams.Solid(27).MoI  MomentsOfInertiaUnits=lbm*in^2  ProductsOfInertia=frontParams.Solid(27).PoI  ProductsOfInertiaUnits=lbm*in^2  BasedOnType=DensityFromFile  Density=1000  DensityUnits=kg/m^3  DoExposeReferenceFrame=on  SerializedFrames=<Frames/>  GraphicType=FromGeometry  MarkerShape=Sphere  MarkerSize=10  GraphicVisPropType=SimpleVisualProperties  GraphicDiffuseColor=frontParams.Solid(27).color  GraphicSpecularColor=[0.5 0.5 0.5 1.0]  GraphicAmbientColor=[0.15 0.15 0.15 1.0]  GraphicEmissiveColor=[0.0 0.0 0.0 1.0]  GraphicShininess=75  GraphicOpacity=frontParams.Solid(27).opacity
  Transform : sm_lib/Frames and Transforms/Rigid Transform  TranslationMethod=Cartesian  TranslationStandardOffset=0  TranslationLengthUnit=in  TranslationStandardAxis=+Z  TranslationCartesianOffset=frontParams.RigidTransform(40).translation  TranslationROffset=0  TranslationROffsetUnits=m  TranslationZOffset=0  TranslationZOffsetUnits=m  TranslationThetaOffset=0  TranslationThetaOffsetUnits=deg  RotationMethod=ArbitraryAxis  RotationAngleUnits=rad  RotationStandardAxis=+Z  RotationAngle=frontParams.RigidTransform(40).angle  RotationArbitraryAxis=frontParams.RigidTransform(40).axis  FollAlignAxisA=+X  BaseAlignAxisA=+Y  FollAlignAxisB=+Y  BaseAlignAxisB=+Z  RotationSequenceAxes=FollowerAxes  RotationSequence=XYX  RotationSequenceAngles=[0 0 0]  RotationSequenceAnglesUnits=deg  RotationMatrix=[1 0 0; 0 1 0; 0 0 1]
  G : PMIOPort  Side=Left
  connections:
  ReferenceFrame/RConn1 -- Solid/RConn1 -- Transform/RConn1
  Transform/LConn1 -- G/RConn1

== system KillerWhaleModel/HeadLinkage/HeadLink1_1/Part_4_1_RIGID ==
  ReferenceFrame : sm_lib/Frames and Transforms/Reference Frame
  Solid : sm_lib/Body Elements/File Solid  ExtGeomFileName=Part 42.step  UnitType=FromFile  ExtGeomFileUnits=m  StepReaderType=HEX  ExportConvexHullGeometry=off  InertiaType=Custom  Mass=frontParams.Solid(29).mass  MassUnits=lbm  CenterOfMass=frontParams.Solid(29).CoM  CenterOfMassUnits=in  MomentsOfInertia=frontParams.Solid(29).MoI  MomentsOfInertiaUnits=lbm*in^2  ProductsOfInertia=frontParams.Solid(29).PoI  ProductsOfInertiaUnits=lbm*in^2  BasedOnType=DensityFromFile  Density=1000  DensityUnits=kg/m^3  DoExposeReferenceFrame=on  SerializedFrames=<Frames/>  GraphicType=FromGeometry  MarkerShape=Sphere  MarkerSize=10  GraphicVisPropType=SimpleVisualProperties  GraphicDiffuseColor=frontParams.Solid(29).color  GraphicSpecularColor=[0.5 0.5 0.5 1.0]  GraphicAmbientColor=[0.15 0.15 0.15 1.0]  GraphicEmissiveColor=[0.0 0.0 0.0 1.0]  GraphicShininess=75  GraphicOpacity=frontParams.Solid(29).opacity
  Transform : sm_lib/Frames and Transforms/Rigid Transform  TranslationMethod=Cartesian  TranslationStandardOffset=0  TranslationLengthUnit=in  TranslationStandardAxis=+Z  TranslationCartesianOffset=frontParams.RigidTransform(42).translation  TranslationROffset=0  TranslationROffsetUnits=m  TranslationZOffset=0  TranslationZOffsetUnits=m  TranslationThetaOffset=0  TranslationThetaOffsetUnits=deg  RotationMethod=ArbitraryAxis  RotationAngleUnits=rad  RotationStandardAxis=+Z  RotationAngle=frontParams.RigidTransform(42).angle  RotationArbitraryAxis=frontParams.RigidTransform(42).axis  FollAlignAxisA=+X  BaseAlignAxisA=+Y  FollAlignAxisB=+Y  BaseAlignAxisB=+Z  RotationSequenceAxes=FollowerAxes  RotationSequence=XYX  RotationSequenceAngles=[0 0 0]  RotationSequenceAnglesUnits=deg  RotationMatrix=[1 0 0; 0 1 0; 0 0 1]
  G : PMIOPort  Side=Left
  connections:
  ReferenceFrame/RConn1 -- Solid/RConn1 -- Transform/RConn1
  Transform/LConn1 -- G/RConn1

== system KillerWhaleModel/HeadLinkage/HeadLink1_1/Part_4_2_RIGID ==
  ReferenceFrame : sm_lib/Frames and Transforms/Reference Frame
  Solid : sm_lib/Body Elements/File Solid  ExtGeomFileName=Part 41.step  UnitType=FromFile  ExtGeomFileUnits=m  StepReaderType=HEX  ExportConvexHullGeometry=off  InertiaType=Custom  Mass=frontParams.Solid(30).mass  MassUnits=lbm  CenterOfMass=frontParams.Solid(30).CoM  CenterOfMassUnits=in  MomentsOfInertia=frontParams.Solid(30).MoI  MomentsOfInertiaUnits=lbm*in^2  ProductsOfInertia=frontParams.Solid(30).PoI  ProductsOfInertiaUnits=lbm*in^2  BasedOnType=DensityFromFile  Density=1000  DensityUnits=kg/m^3  DoExposeReferenceFrame=on  SerializedFrames=<Frames/>  GraphicType=FromGeometry  MarkerShape=Sphere  MarkerSize=10  GraphicVisPropType=SimpleVisualProperties  GraphicDiffuseColor=frontParams.Solid(30).color  GraphicSpecularColor=[0.5 0.5 0.5 1.0]  GraphicAmbientColor=[0.15 0.15 0.15 1.0]  GraphicEmissiveColor=[0.0 0.0 0.0 1.0]  GraphicShininess=75  GraphicOpacity=frontParams.Solid(30).opacity
  Transform : sm_lib/Frames and Transforms/Rigid Transform  TranslationMethod=Cartesian  TranslationStandardOffset=0  TranslationLengthUnit=in  TranslationStandardAxis=+Z  TranslationCartesianOffset=frontParams.RigidTransform(43).translation  TranslationROffset=0  TranslationROffsetUnits=m  TranslationZOffset=0  TranslationZOffsetUnits=m  TranslationThetaOffset=0  TranslationThetaOffsetUnits=deg  RotationMethod=ArbitraryAxis  RotationAngleUnits=rad  RotationStandardAxis=+Z  RotationAngle=frontParams.RigidTransform(43).angle  RotationArbitraryAxis=frontParams.RigidTransform(43).axis  FollAlignAxisA=+X  BaseAlignAxisA=+Y  FollAlignAxisB=+Y  BaseAlignAxisB=+Z  RotationSequenceAxes=FollowerAxes  RotationSequence=XYX  RotationSequenceAngles=[0 0 0]  RotationSequenceAnglesUnits=deg  RotationMatrix=[1 0 0; 0 1 0; 0 0 1]
  G : PMIOPort  Side=Left
  connections:
  ReferenceFrame/RConn1 -- Solid/RConn1 -- Transform/RConn1
  Transform/LConn1 -- G/RConn1

== system KillerWhaleModel/HeadLinkage/HeadLink1_1/Part_5_1_RIGID ==
  ReferenceFrame : sm_lib/Frames and Transforms/Reference Frame
  Solid : sm_lib/Body Elements/File Solid  ExtGeomFileName=Part 51.step  UnitType=FromFile  ExtGeomFileUnits=m  StepReaderType=HEX  ExportConvexHullGeometry=off  InertiaType=Custom  Mass=frontParams.Solid(19).mass  MassUnits=lbm  CenterOfMass=frontParams.Solid(19).CoM  CenterOfMassUnits=in  MomentsOfInertia=frontParams.Solid(19).MoI  MomentsOfInertiaUnits=lbm*in^2  ProductsOfInertia=frontParams.Solid(19).PoI  ProductsOfInertiaUnits=lbm*in^2  BasedOnType=DensityFromFile  Density=1000  DensityUnits=kg/m^3  DoExposeReferenceFrame=on  SerializedFrames=<Frames/>  GraphicType=FromGeometry  MarkerShape=Sphere  MarkerSize=10  GraphicVisPropType=SimpleVisualProperties  GraphicDiffuseColor=frontParams.Solid(19).color  GraphicSpecularColor=[0.5 0.5 0.5 1.0]  GraphicAmbientColor=[0.15 0.15 0.15 1.0]  GraphicEmissiveColor=[0.0 0.0 0.0 1.0]  GraphicShininess=75  GraphicOpacity=frontParams.Solid(19).opacity
  Transform : sm_lib/Frames and Transforms/Rigid Transform  TranslationMethod=Cartesian  TranslationStandardOffset=0  TranslationLengthUnit=in  TranslationStandardAxis=+Z  TranslationCartesianOffset=frontParams.RigidTransform(32).translation  TranslationROffset=0  TranslationROffsetUnits=m  TranslationZOffset=0  TranslationZOffsetUnits=m  TranslationThetaOffset=0  TranslationThetaOffsetUnits=deg  RotationMethod=ArbitraryAxis  RotationAngleUnits=rad  RotationStandardAxis=+Z  RotationAngle=frontParams.RigidTransform(32).angle  RotationArbitraryAxis=frontParams.RigidTransform(32).axis  FollAlignAxisA=+X  BaseAlignAxisA=+Y  FollAlignAxisB=+Y  BaseAlignAxisB=+Z  RotationSequenceAxes=FollowerAxes  RotationSequence=XYX  RotationSequenceAngles=[0 0 0]  RotationSequenceAnglesUnits=deg  RotationMatrix=[1 0 0; 0 1 0; 0 0 1]
  G : PMIOPort  Side=Left
  connections:
  ReferenceFrame/RConn1 -- Solid/RConn1 -- Transform/RConn1
  Transform/LConn1 -- G/RConn1

== system KillerWhaleModel/HeadLinkage/HeadLink1_1/Part_5_2_RIGID ==
  ReferenceFrame : sm_lib/Frames and Transforms/Reference Frame
  Solid : sm_lib/Body Elements/File Solid  ExtGeomFileName=Part 52.step  UnitType=FromFile  ExtGeomFileUnits=m  StepReaderType=HEX  ExportConvexHullGeometry=off  InertiaType=Custom  Mass=frontParams.Solid(8).mass  MassUnits=lbm  CenterOfMass=frontParams.Solid(8).CoM  CenterOfMassUnits=in  MomentsOfInertia=frontParams.Solid(8).MoI  MomentsOfInertiaUnits=lbm*in^2  ProductsOfInertia=frontParams.Solid(8).PoI  ProductsOfInertiaUnits=lbm*in^2  BasedOnType=DensityFromFile  Density=1000  DensityUnits=kg/m^3  DoExposeReferenceFrame=on  SerializedFrames=<Frames/>  GraphicType=FromGeometry  MarkerShape=Sphere  MarkerSize=10  GraphicVisPropType=SimpleVisualProperties  GraphicDiffuseColor=frontParams.Solid(8).color  GraphicSpecularColor=[0.5 0.5 0.5 1.0]  GraphicAmbientColor=[0.15 0.15 0.15 1.0]  GraphicEmissiveColor=[0.0 0.0 0.0 1.0]  GraphicShininess=75  GraphicOpacity=frontParams.Solid(8).opacity
  Transform : sm_lib/Frames and Transforms/Rigid Transform  TranslationMethod=Cartesian  TranslationStandardOffset=0  TranslationLengthUnit=in  TranslationStandardAxis=+Z  TranslationCartesianOffset=frontParams.RigidTransform(21).translation  TranslationROffset=0  TranslationROffsetUnits=m  TranslationZOffset=0  TranslationZOffsetUnits=m  TranslationThetaOffset=0  TranslationThetaOffsetUnits=deg  RotationMethod=ArbitraryAxis  RotationAngleUnits=rad  RotationStandardAxis=+Z  RotationAngle=frontParams.RigidTransform(21).angle  RotationArbitraryAxis=frontParams.RigidTransform(21).axis  FollAlignAxisA=+X  BaseAlignAxisA=+Y  FollAlignAxisB=+Y  BaseAlignAxisB=+Z  RotationSequenceAxes=FollowerAxes  RotationSequence=XYX  RotationSequenceAngles=[0 0 0]  RotationSequenceAnglesUnits=deg  RotationMatrix=[1 0 0; 0 1 0; 0 0 1]
  G : PMIOPort  Side=Left
  connections:
  ReferenceFrame/RConn1 -- Solid/RConn1 -- Transform/RConn1
  Transform/LConn1 -- G/RConn1

== system KillerWhaleModel/HeadLinkage/HeadLink1_1/Part_65_1_RIGID ==
  ReferenceFrame : sm_lib/Frames and Transforms/Reference Frame
  Solid : sm_lib/Body Elements/File Solid  ExtGeomFileName=Part 65.step  UnitType=FromFile  ExtGeomFileUnits=m  StepReaderType=HEX  ExportConvexHullGeometry=off  InertiaType=Custom  Mass=frontParams.Solid(58).mass  MassUnits=lbm  CenterOfMass=frontParams.Solid(58).CoM  CenterOfMassUnits=in  MomentsOfInertia=frontParams.Solid(58).MoI  MomentsOfInertiaUnits=lbm*in^2  ProductsOfInertia=frontParams.Solid(58).PoI  ProductsOfInertiaUnits=lbm*in^2  BasedOnType=DensityFromFile  Density=1000  DensityUnits=kg/m^3  DoExposeReferenceFrame=on  SerializedFrames=<Frames/>  GraphicType=FromGeometry  MarkerShape=Sphere  MarkerSize=10  GraphicVisPropType=SimpleVisualProperties  GraphicDiffuseColor=frontParams.Solid(58).color  GraphicSpecularColor=[0.5 0.5 0.5 1.0]  GraphicAmbientColor=[0.15 0.15 0.15 1.0]  GraphicEmissiveColor=[0.0 0.0 0.0 1.0]  GraphicShininess=75  GraphicOpacity=frontParams.Solid(58).opacity
  Transform : sm_lib/Frames and Transforms/Rigid Transform  TranslationMethod=Cartesian  TranslationStandardOffset=0  TranslationLengthUnit=in  TranslationStandardAxis=+Z  TranslationCartesianOffset=frontParams.RigidTransform(71).translation  TranslationROffset=0  TranslationROffsetUnits=m  TranslationZOffset=0  TranslationZOffsetUnits=m  TranslationThetaOffset=0  TranslationThetaOffsetUnits=deg  RotationMethod=ArbitraryAxis  RotationAngleUnits=rad  RotationStandardAxis=+Z  RotationAngle=frontParams.RigidTransform(71).angle  RotationArbitraryAxis=frontParams.RigidTransform(71).axis  FollAlignAxisA=+X  BaseAlignAxisA=+Y  FollAlignAxisB=+Y  BaseAlignAxisB=+Z  RotationSequenceAxes=FollowerAxes  RotationSequence=XYX  RotationSequenceAngles=[0 0 0]  RotationSequenceAnglesUnits=deg  RotationMatrix=[1 0 0; 0 1 0; 0 0 1]
  G : PMIOPort  Side=Left
  connections:
  ReferenceFrame/RConn1 -- Solid/RConn1 -- Transform/RConn1
  Transform/LConn1 -- G/RConn1
